simulink model "untitled1"  (R2019b)
settings: Solver=VariableStepAuto  StartTime=0.0  StopTime=10.0  RelTol=1e-3
values from neighbouring files (symbols this model uses):
  D = 0.008    [Main.m]
  M = 0.15    [Main.m]
  R = 3    [Main.m]
  Tb = 0.1    [Main.m]
  Td = 5    [Main.m]
  Tg = 0.1    [Main.m]
settings Model: Creator=Asus  LastModifiedBy=Asus

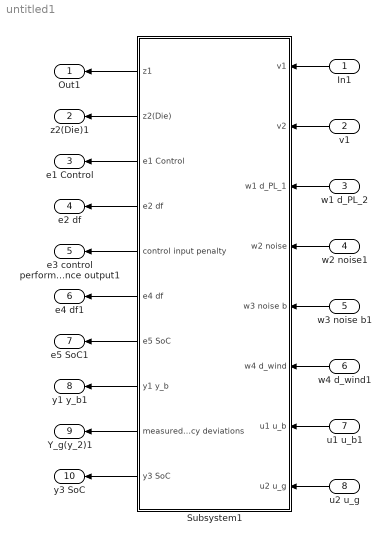
== system untitled1 ==
  In1 : Inport
  v1 : Inport  Port=2
  w1 d_PL_2 : Inport  Port=3
  w2 noise1 : Inport  Port=4
  w3 noise b1 : Inport  Port=5
  w4 d_wind1 : Inport  Port=6
  u1 u_b1 : Inport  Port=7
  "u2 u_g " : Inport  Port=8
  Subsystem1 : Subsystem
  Out1 : Outport
  z2(Die)1 : Outport  Port=2
  e1 Control : Outport  Port=3
  e2 df : Outport  Port=4
  e3 control performance output1 : Outport  Port=5
  e4 df1 : Outport  Port=6
  e5 SoC1 : Outport  Port=7
  y1 y_b1 : Outport  Port=8
  Y_g(y_2)1 : Outport  Port=9
  y3 SoC : Outport  Port=10
  wires:
  Subsystem1/10(y3 SoC) -> y3 SoC/1
  Subsystem1/9(measured frequency deviations) -> Y_g(y_2)1/1
  Subsystem1/7(e5 SoC) -> e5 SoC1/1
  Subsystem1/6(e4 df) -> e4 df1/1
  Subsystem1/5(control input penalty) -> e3 control performance output1/1
  Subsystem1/4(e2 df) -> e2 df/1
  Subsystem1/3(e1 Control) -> e1 Control/1
  "u2 u_g "/1 -> Subsystem1/8("u2 u_g ")
  Subsystem1/1(z1) -> Out1/1
  w4 d_wind1/1 -> Subsystem1/6(w4 d_wind)
  w2 noise1/1 -> Subsystem1/4(w2 noise)
  Subsystem1/2(z2(Die)) -> z2(Die)1/1
  w3 noise b1/1 -> Subsystem1/5(w3 noise b)
  u1 u_b1/1 -> Subsystem1/7(u1 u_b)
  Subsystem1/8(y1 y_b) -> y1 y_b1/1
  v1/1 -> Subsystem1/2(v2)
  w1 d_PL_2/1 -> Subsystem1/3(w1 d_PL_1)
  In1/1 -> Subsystem1/1(v1)

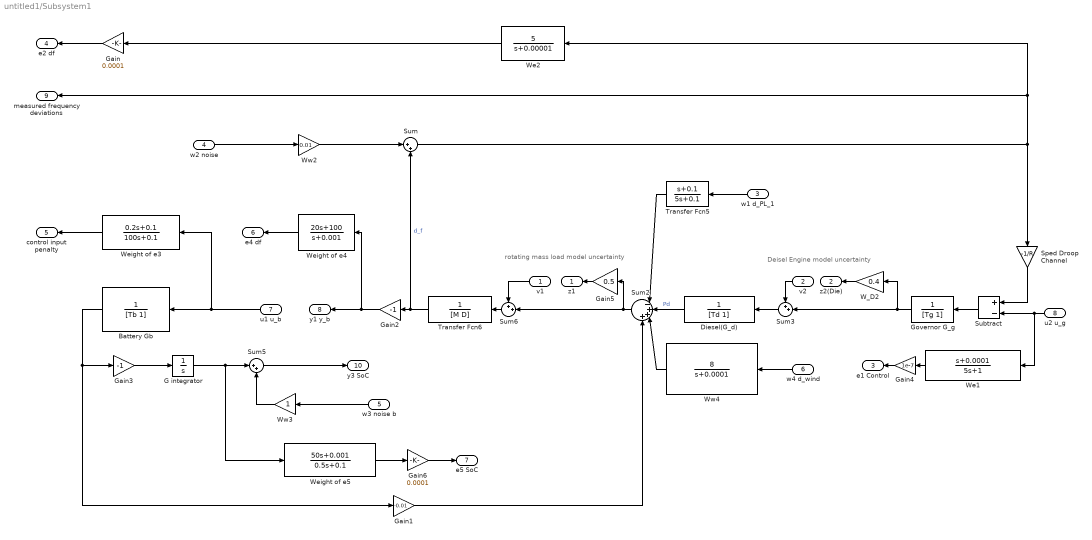
== system untitled1/Subsystem1 ==
  note: Deisel Engine model uncertainty
  note: rotating mass load model
      |                  uncertainty
  v1 : Inport
  v2 : Inport  Port=2
  w1 d_PL_1 : Inport  Port=3
  w2 noise : Inport  Port=4
  w3 noise b : Inport  Port=5
  w4 d_wind : Inport  Port=6
  u1 u_b : Inport  Port=7
  "u2 u_g " : Inport  Port=8
  Battery Gb : TransferFcn  Denominator=[Tb 1]
  Diesel(G_d) : TransferFcn  Denominator=[Td 1]
  "G integrator\t" : Integrator
  Gain : Gain  Gain=0.0001
  Gain1 : Gain  Gain=-0.01
  Gain2 : Gain  Gain=-1
  Gain3 : Gain  Gain=-1
  Gain4 : Gain  Gain=1e-7
  Gain5 : Gain  Gain=0.5
  Gain6 : Gain  Gain=0.0001
  Governor G_g : TransferFcn  Denominator=[Tg 1]
  Sped Droop Channel : Gain  Gain=-1/R
  Subtract : Sum  Inputs=+-
  Sum : Sum  Inputs=|++
  Sum2 : Sum  Inputs=|-+++
  Sum3 : Sum  Inputs=++|
  Sum5 : Sum  Inputs=|++
  Sum6 : Sum  Inputs=++|
  Transfer Fcn5 : TransferFcn  Numerator=[1 0.1]  Denominator=[5 0.1]
  Transfer Fcn6 : TransferFcn  Denominator=[M D]
  W_D2 : Gain  Gain=0.4
  We1 : TransferFcn  Numerator=[1 0.0001]  Denominator=[5 1]
  We2 : TransferFcn  Numerator=[5]  Denominator=[1 0.00001]
  Weight of e3 : TransferFcn  Numerator=[0.2 0.1]  Denominator=[100 0.1]
  Weight of e4 : TransferFcn  Numerator=[20 100]  Denominator=[1 0.001]
  Weight of e5 : TransferFcn  Numerator=[50 0.001]  Denominator=[0.5 0.1]
  Ww2 : Gain  Gain=0.01
  Ww3 : Gain
  Ww4 : TransferFcn  Numerator=[8]  Denominator=[1 0.0001]
  z1 : Outport
  z2(Die) : Outport  Port=2
  e1 Control : Outport  Port=3
  e2 df : Outport  Port=4
  control input penalty : Outport  Port=5
  e4 df : Outport  Port=6
  e5 SoC : Outport  Port=7
  y1 y_b : Outport  Port=8
  measured frequency deviations : Outport  Port=9
  y3 SoC : Outport  Port=10
  wires:
  v2/1 -> Sum3/1
  v1/1 -> Sum6/1
  w2 noise/1 -> Ww2/1
  Transfer Fcn6/1 -> Sum/2, Gain2/1  "d_f"
  "G integrator\t"/1 -> Weight of e5/1, Sum5/1
  Gain2/1 -> Weight of e4/1, y1 y_b/1
  Ww2/1 -> Sum/1
  w3 noise b/1 -> Ww3/1
  Subtract/1 -> Governor G_g/1
  w4 d_wind/1 -> Ww4/1
  "u2 u_g "/1 -> We1/1, Subtract/2
  u1 u_b/1 -> Weight of e3/1, Battery Gb/1
  w1 d_PL_1/1 -> Transfer Fcn5/1
  Gain5/1 -> z1/1
  Sum/1 -> We2/1, measured frequency deviations/1, Sped Droop Channel/1
  Ww4/1 -> Sum2/3
  W_D2/1 -> z2(Die)/1
  Sum5/1 -> y3 SoC/1
  Sum2/1 -> Gain5/1, Sum6/2
  Diesel(G_d)/1 -> Sum2/2  "Pd"
  Gain1/1 -> Sum2/4
  Gain3/1 -> "G integrator\t"/1
  Sum3/1 -> Diesel(G_d)/1
  Sped Droop Channel/1 -> Subtract/1
  Transfer Fcn5/1 -> Sum2/1
  Governor G_g/1 -> Sum3/2, W_D2/1
  Battery Gb/1 -> Gain1/1, Gain3/1
  Ww3/1 -> Sum5/2
  Sum6/1 -> Transfer Fcn6/1
  Gain/1 -> e2 df/1
  We2/1 -> Gain/1
  Gain4/1 -> e1 Control/1
  We1/1 -> Gain4/1
  Weight of e5/1 -> Gain6/1
  Gain6/1 -> e5 SoC/1
  Weight of e3/1 -> control input penalty/1
  Weight of e4/1 -> e4 df/1
